simulink model "Explicit_MPC_Controller"  (R2024b)
settings: configuration reference "linear_controller_config" (kept outside this file)
libraries: mpclib x1
settings Model: DataDictionary=sim_data_DCmotor_system.sldd  Creator=tshintai  LastModifiedBy=tshintai
settings ConfigSetRef: SourceName=linear_controller_config

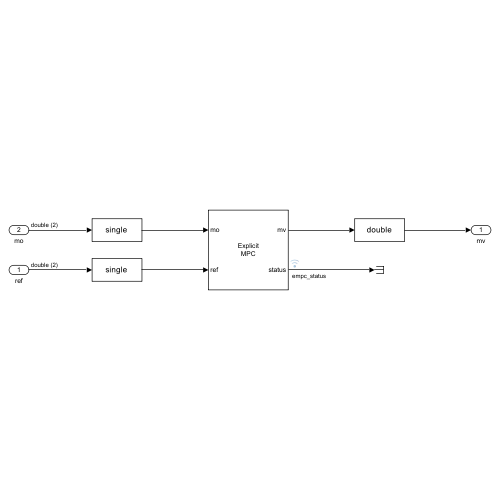
[thumbnail: Simulink's stored preview of the top-level diagram]
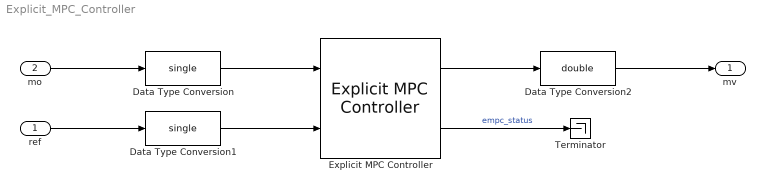
== system Explicit_MPC_Controller ==
  ref : Inport  OutDataTypeStr=double  PortDimensions=2
  mo : Inport  Port=2  OutDataTypeStr=double  PortDimensions=2
  Data Type Conversion : DataTypeConversion  OutDataTypeStr=single  SaturateOnIntegerOverflow=off  RndMeth=Floor
  Data Type Conversion1 : DataTypeConversion  OutDataTypeStr=single  SaturateOnIntegerOverflow=off  RndMeth=Floor
  Data Type Conversion2 : DataTypeConversion  OutDataTypeStr=double  SaturateOnIntegerOverflow=off  RndMeth=Floor
  Explicit MPC Controller : mpclib/Explicit MPC Controller  SCDEnableBlockLinearizationSpecification=on  empcobj=mpcObjExplicit  x0=[]  is_multiple=0  enable_value=0  return_u0=off  md_inport=off  mv_inport=off  return_status=on  return_region=off  return_state=off  state_inport=off  BlockDataType=single  SampleTimeInherited=off  switch_inport=off
  Terminator : Terminator
  mv : Outport
  wires:
  Data Type Conversion1/1 -> Explicit MPC Controller/2
  Explicit MPC Controller/1 -> Data Type Conversion2/1
  ref/1 -> Data Type Conversion1/1
  Data Type Conversion2/1 -> mv/1
  Data Type Conversion/1 -> Explicit MPC Controller/1
  mo/1 -> Data Type Conversion/1
  Explicit MPC Controller/2 -> Terminator/1  "empc_status"
